simulink model "StateSpaceControllerNominal"  (R2020b)
settings: Solver=ode45  StartTime=0.0  StopTime=30  MaxStep=0.001  RelTol=1e-3
settings Model: Creator=umberto  LastModifiedBy=Musta

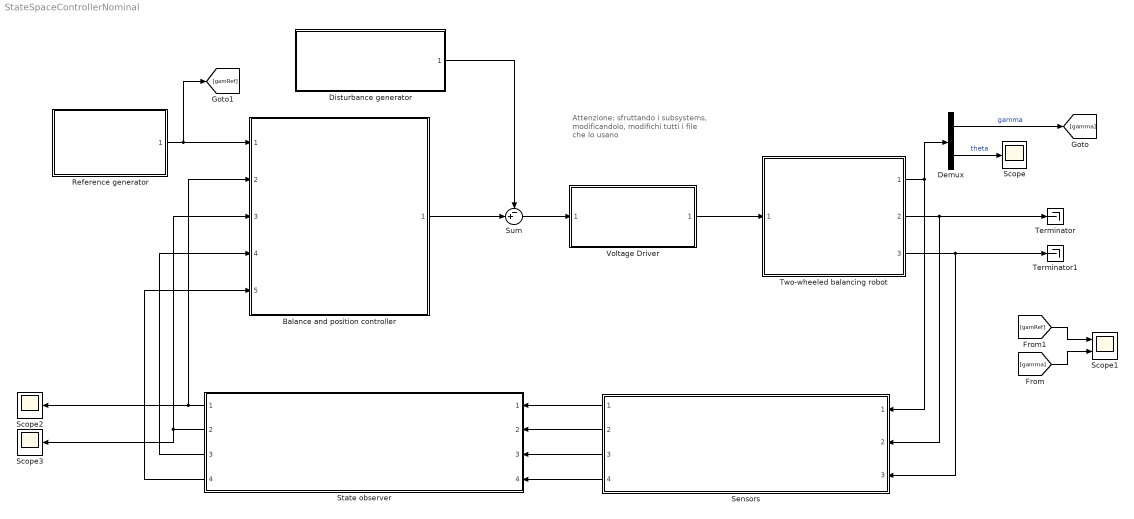
== system StateSpaceControllerNominal ==
  note: Attenzione: sfruttando i subsystems, modificandolo, modifichi tutti i file che lo usano
  Balance and position controller : Subsystem  ReferencedSubsystem=StateSpaceControllerNominal_SubSystem
  Demux : Demux  Outputs=2
  Disturbance generator : Subsystem  ReferencedSubsystem=DisturbanceGenerator_SubSystem
  Reference generator : Subsystem  ReferencedSubsystem=GeneratorGam_ref_SubSystem
  Scope : Scope
  Scope1 : Scope  NumInputPorts=2
  Scope2 : Scope
  Scope3 : Scope
  Sensors : Subsystem  ReferencedSubsystem=Sensors_SubSystem
      settings: PortSchema="{\"entries\":[{\"content\":{\"sides\":[{\"content\":{\"connectorIds\":[\"Out1\",\"Out2\",\"Out3\",\"Out4\"]},\"type\":\"ConnectorPlacement.EquallySpacedRectSide\",\"uuid\":\"51d9aeda-2f58-468a-8445-73d257530b17\"},{\"content\":{\"connectorIds\":[\"In1\",\"In2\",\"In3\"],\"side\":\"RIGHT\"},\"type\":\"ConnectorPlacement.EquallySpacedRectSide\",\"uuid\":\"77571700-4d1b-47e5-9f8b-52ba036b938f\"},{\"content\":{\"connectorIds\":[],\"side\":\"TOP\"},\"type\":\"ConnectorPlacement.EquallySpacedRectSide\",\"uuid\":\"3da4c363-45f4-4830-b4e0-aa9f00660111\"},{\"content\":{\"connectorIds\":[],\"side\":\"HIDDEN\"},\"type\":\"ConnectorPlacement.EquallySpacedRectSide\",\"uuid\":\"a0dec54f-3332-4ba1-b47c-c34ae4f51399\"}]},\"type\":\"ConnectorPlacement.EquallySpacedConnector\",\"uuid\":\"468e00a1-da97-4578-a7a9-89bb9365fd7e\"}],\"packageUris\":[\"http://schema.mathworks.com/mf0/Connector/R2020b\"],\"version\":\"1.0\"}"
  State observer : Subsystem  ReferencedSubsystem=SimpleStateObserver_SubSystem
  Sum : Sum  Inputs=-+|
  Terminator : Terminator
  Terminator1 : Terminator
  Two-wheeled balancing robot : Subsystem  ReferencedSubsystem=Robot_SubSystem
  Voltage Driver : Subsystem  ReferencedSubsystem=VoltageDriver_SubSystem
  wires:
  State observer/1 -> Scope2/1, Balance and position controller/2
  State observer/2 -> Scope3/1, Balance and position controller/3
  State observer/3 -> Balance and position controller/4
  State observer/4 -> Balance and position controller/5
  Two-wheeled balancing robot/1 -> Sensors/1, Demux/1
  Demux/2 -> Scope/1  "theta"
  Demux/1 -> [gamma]  "gamma"
  Reference generator/1 -> [gamRef], Balance and position controller/1
  Balance and position controller/1 -> Sum/2
  Sum/1 -> Voltage Driver/1
  Disturbance generator/1 -> Sum/1
  Voltage Driver/1 -> Two-wheeled balancing robot/1
  Two-wheeled balancing robot/2 -> Sensors/2, Terminator/1
  Two-wheeled balancing robot/3 -> Sensors/3, Terminator1/1
  Sensors/1 -> State observer/1
  Sensors/2 -> State observer/2
  Sensors/3 -> State observer/3
  Sensors/4 -> State observer/4
  [gamRef] -> Scope1/1
  [gamma] -> Scope1/2
